simulink model "MATE_SwitchedReluctanceMotor64Drive"  (R2024b)
settings: Solver=FixedStepDiscrete  StartTime=0.0  StopTime=5  FixedStep=Ts  RelTol=1e-3  AbsTol=1e-5  EnableMultiTasking=on
PreLoadFcn:
  | Ts=1e-6;Rsnu=100; Csnu=1e-6;
  | 
  | % Magnetisation characteristic table of the switched Reluctance Motor:
  | % Table elements =  Flux linkage, in Wb.
  | 
  | FluxTable = [
  |     0             0              0             0             0             0
  |     0.3220    0.3050    0.2280    0.1240    0.0220    0.0170
  |     0.3760    0.3570    0.2770    0.1600    0.0420    0.0340
  |     0.3990    0.3850    0.3000    0.1830    0.0640    0.0500
  |     0.4160    0.4020    0.3200    0.2010    0.0840    0.0670
  |     0.4280    0.4150    0.3340    0.2190    0.1030    0.0840
  |     0.4370    0.4260    0.3480    0.2370    0.1230    0.1010
  |     0.4430    0.4330    0.3590    0.2530    0.1420    0.1170
  |     0.4490    0.4390    0.3710    0.2680    0.1610    0.1340
  |     0.4540    0.4440    0.3820    0.2820    0.1790    0.1510
  |     0.4590    0.4490    0.3920    0.2950    0.1970    0.1680
  |     0.4630    0.4530    0.4020    0.3090    0.2140    0.1840
  |     0.4670    0.4570    0.4110    0.3220    0.2310    0.2010
  |     0.4700    0.4620    0.4190    0.3360    0.2460    0.2180
  |     0.4740    0.4650    0.4270    0.3480    0.2610    0.2350
  |     0.4780    0.4690    0.4330    0.3590    0.2770    0.2510
  |     0.4810    0.4730    0.4380    0.3690    0.2910    0.2680
  |     0.4840    0.4770    0.4440    0.3800    0.3050    0.2850
  |     0.4870    0.4790    0.4480    0.3890    0.3200    0.3020];
  | 
  | % Table columns :  Rotor angles, in degrees.
  | 
  | RotorAngles = [
  |     0             10            20            30            40            45];
  | 
  | % Table rows : Stator current, in A.
  | 
  | StatorCurrents = [ 0:size(FluxTable,1)-1] * 25;
PostLoadFcn:
  | Ts=1e-6;Rsnu=100; Csnu=1e-6;
  | 
  | % Magnetisation characteristic table of the switched Reluctance Motor:
  | % Table elements =  Flux linkage, in Wb.
  | 
  | FluxTable = [
  |     0             0              0             0             0             0
  |     0.3220    0.3050    0.2280    0.1240    0.0220    0.0170
  |     0.3760    0.3570    0.2770    0.1600    0.0420    0.0340
  |     0.3990    0.3850    0.3000    0.1830    0.0640    0.0500
  |     0.4160    0.4020    0.3200    0.2010    0.0840    0.0670
  |     0.4280    0.4150    0.3340    0.2190    0.1030    0.0840
  |     0.4370    0.4260    0.3480    0.2370    0.1230    0.1010
  |     0.4430    0.4330    0.3590    0.2530    0.1420    0.1170
  |     0.4490    0.4390    0.3710    0.2680    0.1610    0.1340
  |     0.4540    0.4440    0.3820    0.2820    0.1790    0.1510
  |     0.4590    0.4490    0.3920    0.2950    0.1970    0.1680
  |     0.4630    0.4530    0.4020    0.3090    0.2140    0.1840
  |     0.4670    0.4570    0.4110    0.3220    0.2310    0.2010
  |     0.4700    0.4620    0.4190    0.3360    0.2460    0.2180
  |     0.4740    0.4650    0.4270    0.3480    0.2610    0.2350
  |     0.4780    0.4690    0.4330    0.3590    0.2770    0.2510
  |     0.4810    0.4730    0.4380    0.3690    0.2910    0.2680
  |     0.4840    0.4770    0.4440    0.3800    0.3050    0.2850
  |     0.4870    0.4790    0.4480    0.3890    0.3200    0.3020];
  | 
  | % Table columns :  Rotor angles, in degrees.
  | 
  | RotorAngles = [
  |     0             10            20            30            40            45];
  | 
  | % Table rows : Stator current, in A.
  | 
  | StatorCurrents = [ 0:size(FluxTable,1)-1] * 25;
InitFcn:
  | Ts=1e-6;Rsnu=100; Csnu=1e-6;
  | 
  | % Magnetisation characteristic table of the switched Reluctance Motor:
  | % Table elements =  Flux linkage, in Wb.
  | 
  | FluxTable = [
  |     0             0              0             0             0             0
  |     0.3220    0.3050    0.2280    0.1240    0.0220    0.0170
  |     0.3760    0.3570    0.2770    0.1600    0.0420    0.0340
  |     0.3990    0.3850    0.3000    0.1830    0.0640    0.0500
  |     0.4160    0.4020    0.3200    0.2010    0.0840    0.0670
  |     0.4280    0.4150    0.3340    0.2190    0.1030    0.0840
  |     0.4370    0.4260    0.3480    0.2370    0.1230    0.1010
  |     0.4430    0.4330    0.3590    0.2530    0.1420    0.1170
  |     0.4490    0.4390    0.3710    0.2680    0.1610    0.1340
  |     0.4540    0.4440    0.3820    0.2820    0.1790    0.1510
  |     0.4590    0.4490    0.3920    0.2950    0.1970    0.1680
  |     0.4630    0.4530    0.4020    0.3090    0.2140    0.1840
  |     0.4670    0.4570    0.4110    0.3220    0.2310    0.2010
  |     0.4700    0.4620    0.4190    0.3360    0.2460    0.2180
  |     0.4740    0.4650    0.4270    0.3480    0.2610    0.2350
  |     0.4780    0.4690    0.4330    0.3590    0.2770    0.2510
  |     0.4810    0.4730    0.4380    0.3690    0.2910    0.2680
  |     0.4840    0.4770    0.4440    0.3800    0.3050    0.2850
  |     0.4870    0.4790    0.4480    0.3890    0.3200    0.3020];
  | 
  | % Table columns :  Rotor angles, in degrees.
  | 
  | RotorAngles = [
  |     0             10            20            30            40            45];
  | 
  | % Table rows : Stator current, in A.
  | 
  | StatorCurrents = [ 0:size(FluxTable,1)-1] * 25;
undefined symbols (not defined in the file or in its folder): DiscIntNeverNeededParam
libraries: simetranss x5, fl_lib x3, nesl_utility x2
Description:
  | Copyright 2008-2017 The MathWorks, Inc.
settings Model: ARTEMISmethode_block_infos=$$__separator__$$  Creator=Kyle Diller  LastModifiedBy=CD8435
settings SolverCC: AutoScaleAbsTol=off  AlgebraicLoopSolver=TrustRegion  InsertRTBMode=Auto
settings DataIOCC: LimitDataPoints=on  SaveFormat=Array  SignalLoggingSaveFormat=ModelDataLogs  ReturnWorkspaceOutputs=off  SignalLoggingName=sigsOut
settings OptimizationCC: ExpressionDepthLimit=2147483647  InitFltsAndDblsToZero=on  LifeSpan=inf
settings DebuggingCC: UnderspecifiedInitializationDetection=Classic  MergeDetectMultiDrivingBlocksExec=none  CheckExecutionContextPreStartOutputMsg=on  SignalResolutionControl=TryResolveAllWithWarning  MultiTaskDSMMsg=warning  MultiTaskCondExecSysMsg=none  FcnCallInpInsideContextMsg=warning  UnconnectedInputMsg=warning  UnconnectedOutputMsg=warning  UnconnectedLineMsg=warning  StateNameClashWarn=warning  SFUnexpectedBacktrackingDiag=warning  SFNoUnconditionalDefaultTransitionDiag=warning  SFExecutionAtInitializationDiag=none  ArithmeticOperatorsInVariantConditions=warning
settings HardwareCC: ProdBitPerPointer=32  ProdBitPerSizeT=32  ProdBitPerPtrDiffT=32  ProdLargestAtomicFloat=None  ProdIntDivRoundTo=Undefined  ProdEndianess=Unspecified  ProdWordSize=32  ProdHWDeviceType=32-bit Generic  TargetUnknown=on
settings ModelReferenceCC: EnableRefExpFcnMdlSchedulingChecks=on  PropagateSignalLabelsOutOfModel=off
settings SFSimCC: SimUseLocalCustomCode=off  CustomCodeUndefinedFunction=UseInterfaceOnly
settings RTWCC: RTWUseLocalCustomCode=off  GPUComputeCapability=3.5
settings CodeAppCC: StateflowObjectComments=on
settings GRTTargetCC: TargetLangStandard=C89/C90 (ANSI)  CombineOutputUpdateFcns=off  GRTInterface=on
settings ConfigComp: CovMetricSettings=dw  CovSaveCumulativeToWorkspaceVar=on  CovSaveSingleToWorkspaceVar=on  CovExternalEMLEnable=off  CovSFcnEnable=off
settings SimscapeCC: SimscapeNormalizeSystem=off

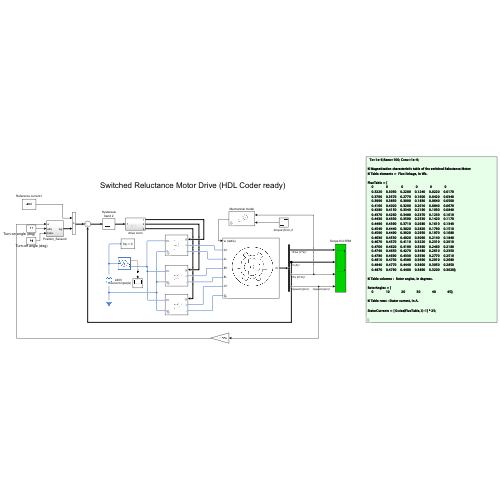
[thumbnail: Simulink's stored preview of the top-level diagram]
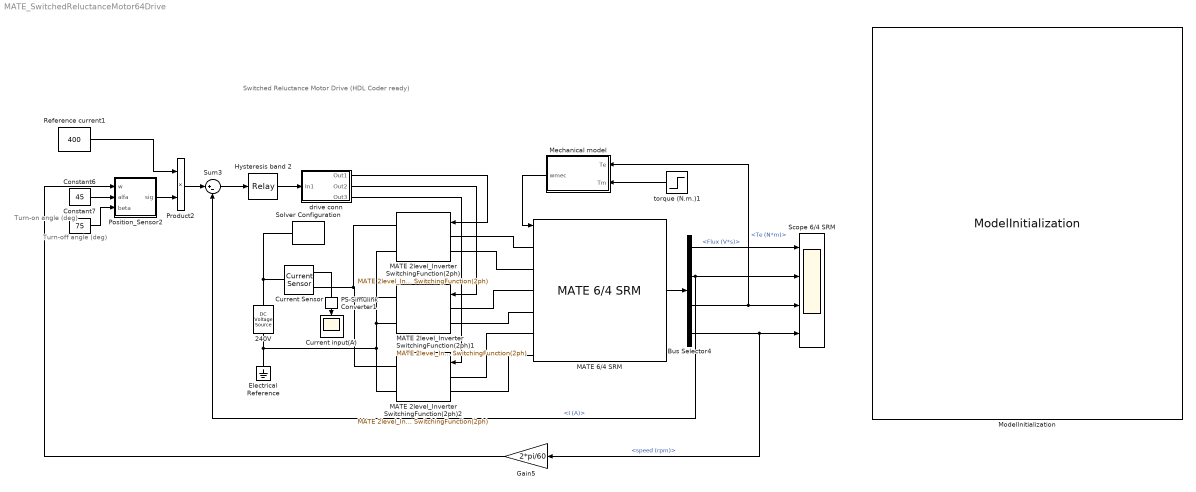
== system MATE_SwitchedReluctanceMotor64Drive ==
  note: Switched Reluctance Motor Drive (HDL Coder ready)
  note: Turn-off angle (deg)
  note: Turn-on angle (deg)
  240V : fl_lib/Electrical/Electrical Sources/DC Voltage Source  v0=240 V
  Bus Selector4 : BusSelector  OutputSignals=Flux (V*s),I (A),Te (N*m),speed (rpm)
  Constant6 : Constant  Value=45
  Constant7 : Constant  Value=75
  Current Sensor : fl_lib/Electrical/Electrical Sensors/Current Sensor
  Current input(A) : Scope
  Electrical Reference : fl_lib/Electrical/Electrical Elements/Electrical Reference
  Gain5 : Gain  Gain=2*pi/60  SaturateOnIntegerOverflow=on  OutDataTypeStr=Inherit: Same as input  ParamDataTypeStr=Inherit: Same as input
  Hysteresis band 2 : Relay  OnSwitchValue=10  OffSwitchValue=-10  SampleTime=Ts
  MATE 2level_Inverter SwitchingFunction(2ph) : simetranss/FPGA/MATE 2level_Inverter  SwitchingFunction(2ph)  Ron=1e-3  Gp=250  Gi=0.1e-6  Ts=Ts  min_charge=0
  MATE 2level_Inverter SwitchingFunction(2ph)1 : simetranss/FPGA/MATE 2level_Inverter  SwitchingFunction(2ph)  Ron=1e-3  Gp=250  Gi=0.1e-6  Ts=Ts  min_charge=0
  MATE 2level_Inverter SwitchingFunction(2ph)2 : simetranss/FPGA/MATE 2level_Inverter  SwitchingFunction(2ph)  Ron=1e-3  Gp=250  Gi=0.1e-6  Ts=Ts  min_charge=0
  MATE 6/4 SRM : simetranss/Machines/MATE 6//4 SRM  MachineType=6/4  Rs=0.05  Inertia=0.05  FluxTable=FluxTable  RotorAngles=RotorAngles  StatorCurrents=StatorCurrents  Friction=0.02  Initialangle=0  TsBlock=-1  nb_points=[100,20,20]  PlotCurves=on
  Mechanical model : Subsystem  mask(Machine rotational mechanical model){J=0.5, F=0.02, fo=0, Ts=Ts}
      mask prompts: J "Inertia (kg.m^2)"; F "Friction (N.m.s)"; fo "Initial mechanical frequency (Hz)"; Ts "Sample Time (s)"
      mask help:
      | This block can implement a simple rotating mechanical equation for machines
      |
      | The block working equation is:
      | wmec=1/J*INT{( Te - Tm -F*wmec )*dt}
      |
      | All values in SI.
      |
      | Parameters:
      | Inertia J (kg.m^2)
      | Friction F (N.m.s)
      | Initial mechanical frequency (Hz)
      | Sample Time (s).
      |
      | Signals:
      | Te: electric torque input from the machine (N.m.)
      | Tm : mechanical torque applied to the shaft (N.m.)
      | wmec: mechanical speed of machine (rad/s)
      |
      | Conversion from Per-Unit values
      |
      | J=2*H*Pn/w_mec^2
      | F=D*Pn/w_mec^2
      | where:
      | J is the inertia in km.m^2
      | H is the inertia constant in seconds.
      | F is the friction factor in N.m.s
      | D in the friction factor or damping factor in pu.
      | Pn is the nominal power of the machine
      | w_mec is the nominal mechanical rotational frequency of the machine in rad/s
  ModelInitialization : simetranss/Usefulls/ModelInitialization  InitFcnX=|  prel=on  posl=on  inif=on  strf=off
      | Ts=1e-6;Rsnu=100; Csnu=1e-6; 
      | 
      | % Magnetisation characteristic table of the switched Reluctance Motor:
      | % Table elements =  Flux linkage, in Wb.
      | 
      | FluxTable = [
      |     0             0              0             0             0             0
      |     0.3220    0.3050    0.2280    0.1240    0.0220    0.0170
      |     0.3760    0.3570    0.2770    0.1600    0.0420    0.0340
      |     0.3990    0.3850    0.3000    0.1830    0.0640    0.0500
      |     0.4160    0.4020    0.3200    0.2010    0.0840    0.0670
      |     0.4280    0.4150    0.3340    0.2190    0.1030    0.0840
      |     0.4370    0.4260    0.3480    0.2370    0.1230    0.1010
      |     0.4430    0.4330    0.3590    0.2530    0.1420    0.1170
      |     0.4490    0.4390    0.3710    0.2680    0.1610    0.1340
      |     0.4540    0.4440    0.3820    0.2820    0.1790    0.1510
      |     0.4590    0.4490    0.3920    0.2950    0.1970    0.1680
      |     0.4630    0.4530    0.4020    0.3090    0.2140    0.1840
      |     0.4670    0.4570    0.4110    0.3220    0.2310    0.2010
      |     0.4700    0.4620    0.4190    0.3360    0.2460    0.2180
      |     0.4740    0.4650    0.4270    0.3480    0.2610    0.2350
      |     0.4780    0.4690    0.4330    0.3590    0.2770    0.2510
      |     0.4810    0.4730    0.4380    0.3690    0.2910    0.2680
      |     0.4840    0.4770    0.4440    0.3800    0.3050    0.2850
      |     0.4870    0.4790    0.4480    0.3890    0.3200    0.3020]; 
      | 
      | % Table columns :  Rotor angles, in degrees.
      | 
      | RotorAngles = [
      |     0             10            20            30            40            45];
      | 
      | % Table rows : Stator current, in A.
      | 
      | StatorCurrents = [ 0:size(FluxTable,1)-1] * 25;
  PS-Simulink Converter1 : nesl_utility/PS-Simulink Converter  PhysicalDomain=network_engine_domain  SubClassName=ps_output  LeftPortType=input  RightPortType=output  PseudoPeriodic=off  Frequencies=[]  VectorFormat=inherit  Unit=inherit  AffineConversion=off
  Position_Sensor2 : Subsystem
  Product2 : Product  SaturateOnIntegerOverflow=on  OutDataTypeStr=Inherit: Same as first input
  Reference current1 : Constant  Value=400
  Scope 6/4 SRM : Scope  NumInputPorts=4
  Solver Configuration : nesl_utility/Solver Configuration  PhysicalDomain=network_engine_domain  SubClassName=solver  LeftPortType=input  RightPortType=generic  Tones=[]  Harmonics=[]  SimulateNoise=off  Profile=off  UseLocalSampling=off  EnableSwitchedLinearOptims=on  FrequencyDomain=off  UseCCode=off  RelTol=0.001  AbsTol=0.001  MinStep=1e-09  ToWorkspace=off  RevertToSquareIcSolve=off  NumHomotopyIterations=100  PhasorMode=off  PhasorModeNumHarmonics=1  ConsistencySolver=NEWTON_XTOL_AFTER_FTOL  IndexReductionMethod=DerivativeReplacement  DoDC=off  ResidualTolerance=1e-09  ConsistencyTolSource=GLOBAL  ConsistencyAbsTol=0.001  ConsistencyRelTol=0.001  ConsistencyTolFactor=0.001  UseLocalSolver=on  LocalSolverChoice=NE_BACKWARD_EULER_ADVANCER  ResolveIndetEquations=on  FunctionEvalNumThread=1  LocalSolverSampleTime=Ts  DoFixedCost=on  MaxNonlinIter=1  MaxModeIter=2  ComputeImpulses=off  ImpulseIterations=2  LinearAlgebra=auto  LinearAlgebraNumThread=0  EquationFormulation=NE_TIME_EF  DelaysMemoryBudget=1024  AutomaticFiltering=on  FilteringTimeConstant=0.001  PartitionStorageMethod=AS_NEEDED  PartitionMemoryBudget=1024  PartitionMethod=ROBUST  MultibodyUseLocalSolver=off  MultibodyLocalSolverChoice=ODE1  MultibodyLocalSolverSampleTime=0.001
  Sum3 : Sum  Inputs=|+-  SaturateOnIntegerOverflow=on
  drive conn : Subsystem
  torque (N.m.)1 : Step  After=100  SampleTime=0
  wires:
  Bus Selector4/3 -> Mechanical model/1(Te), Scope 6/4 SRM/3  "<Te (N*m)>"
  Constant6/1 -> Position_Sensor2/2(alfa)
  Constant7/1 -> Position_Sensor2/3(beta)
  Sum3/1 -> Hysteresis band 2/1
  Product2/1 -> Sum3/1
  Position_Sensor2/1(sig) -> Product2/2
  MATE 6/4 SRM/1 -> Bus Selector4/1
  Bus Selector4/1 -> Scope 6/4 SRM/1  "<Flux (V*s)>"
  Bus Selector4/2 -> Scope 6/4 SRM/2, Sum3/2  "<I (A)>"
  Bus Selector4/4 -> Scope 6/4 SRM/4, Gain5/1  "<speed (rpm)>"
  torque (N.m.)1/1 -> Mechanical model/2(Tm)
  Gain5/1 -> Position_Sensor2/1(w)
  Mechanical model/1(wmec) -> MATE 6/4 SRM/1
  Reference current1/1 -> Product2/1
  drive conn/1(Out1) -> MATE 2level_Inverter SwitchingFunction(2ph)/1
  drive conn/2(Out2) -> MATE 2level_Inverter SwitchingFunction(2ph)1/1
  drive conn/3(Out3) -> MATE 2level_Inverter SwitchingFunction(2ph)2/1
  PS-Simulink Converter1/1 -> Current input(A)/1
  Hysteresis band 2/1 -> drive conn/1(In1)
  connections:
  Solver Configuration/RConn1 -- 240V/LConn1 -- Current Sensor/LConn1
  240V/RConn1 -- MATE 2level_Inverter SwitchingFunction(2ph)2/RConn2 -- MATE 2level_Inverter SwitchingFunction(2ph)1/RConn2 -- MATE 2level_Inverter SwitchingFunction(2ph)/RConn2 -- Electrical Reference/LConn1
  Current Sensor/RConn1 -- PS-Simulink Converter1/LConn1
  MATE 2level_Inverter SwitchingFunction(2ph)2/RConn1 -- MATE 2level_Inverter SwitchingFunction(2ph)1/RConn1 -- MATE 2level_Inverter SwitchingFunction(2ph)/RConn1 -- Current Sensor/RConn2
  MATE 2level_Inverter SwitchingFunction(2ph)/LConn1 -- MATE 6/4 SRM/LConn1
  MATE 2level_Inverter SwitchingFunction(2ph)1/LConn2 -- MATE 6/4 SRM/LConn4
  MATE 2level_Inverter SwitchingFunction(2ph)/LConn2 -- MATE 6/4 SRM/LConn2
  MATE 2level_Inverter SwitchingFunction(2ph)1/LConn1 -- MATE 6/4 SRM/LConn3
  MATE 2level_Inverter SwitchingFunction(2ph)2/LConn2 -- MATE 6/4 SRM/LConn6
  MATE 2level_Inverter SwitchingFunction(2ph)2/LConn1 -- MATE 6/4 SRM/LConn5

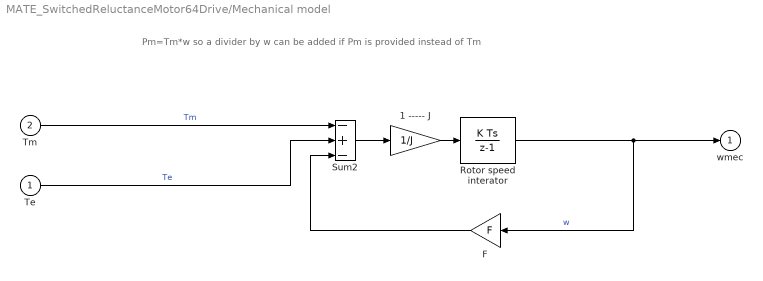
== system MATE_SwitchedReluctanceMotor64Drive/Mechanical model ==
  note: Pm=Tm*w so a divider by w can be added if Pm is provided instead of Tm
  Te : Inport  PortDimensions=1
  Tm : Inport  Port=2
  1 ----- J : Gain  Gain=1/J  SaturateOnIntegerOverflow=on  OutDataTypeStr=Inherit: Same as input  ParamDataTypeStr=Inherit: Same as input
  F : Gain  Gain=F  SaturateOnIntegerOverflow=on  OutDataTypeStr=Inherit: Same as input  ParamDataTypeStr=Inherit: Same as input
  Rotor speed interator : DiscreteIntegrator  InitialCondition=fo*2*pi  SampleTime=Ts  ICPrevOutput=DiscIntNeverNeededParam  ICPrevScaledInput=DiscIntNeverNeededParam
  Sum2 : Sum  Inputs=-+-  InputSameDT=on  SaturateOnIntegerOverflow=on  OutDataTypeStr=Inherit: Same as first input
  wmec : Outport  InitialOutput=0  VectorParamsAs1DForOutWhenUnconnected=off
  wires:
  Tm/1 -> Sum2/1  "Tm"
  Sum2/1 -> 1 ----- J/1
  F/1 -> Sum2/3
  Te/1 -> Sum2/2  "Te"
  1 ----- J/1 -> Rotor speed interator/1
  Rotor speed interator/1 -> wmec/1, F/1  "w"

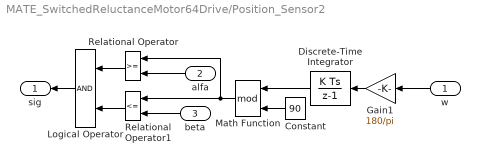
== system MATE_SwitchedReluctanceMotor64Drive/Position_Sensor2 ==
  w : Inport
  alfa : Inport  Port=2
  beta : Inport  Port=3
  Constant : Constant  Value=90
  Discrete-Time Integrator : DiscreteIntegrator  InitialCondition=[0 -30 -60]  SampleTime=Ts  ICPrevOutput=DiscIntNeverNeededParam  ICPrevScaledInput=DiscIntNeverNeededParam
  Gain1 : Gain  Gain=180/pi  SaturateOnIntegerOverflow=on  OutDataTypeStr=Inherit: Same as input  ParamDataTypeStr=Inherit: Same as input
  Logical Operator : Logic  AllPortsSameDT=off
  Math Function : Math  Operator=mod  SignedPower=on
  Relational Operator : RelationalOperator  InputSameDT=off
  Relational Operator1 : RelationalOperator  Operator=<=  InputSameDT=off
  sig : Outport  VectorParamsAs1DForOutWhenUnconnected=off
  wires:
  Logical Operator/1 -> sig/1
  w/1 -> Gain1/1
  Math Function/1 -> Relational Operator/1, Relational Operator1/1
  Relational Operator1/1 -> Logical Operator/2
  Gain1/1 -> Discrete-Time Integrator/1
  beta/1 -> Relational Operator1/2
  alfa/1 -> Relational Operator/2
  Relational Operator/1 -> Logical Operator/1
  Constant/1 -> Math Function/2
  Discrete-Time Integrator/1 -> Math Function/1

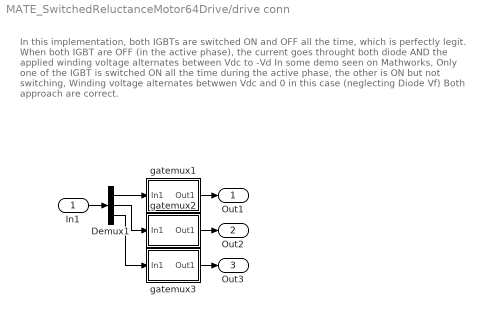
== system MATE_SwitchedReluctanceMotor64Drive/drive conn ==
  note: In this implementation, both IGBTs are switched ON and OFF all the time, which is perfectly legit. When both IGBT are OFF (in the active phase), the current goes throught both diode AND the applied winding voltage alternates between Vdc to -Vd
      |
      | In some demo seen on Mathworks, Only one of the IGBT is switched ON all the time during the active phase, the other is ON but not switching, Winding voltage alternates betwwen Vdc and 0 in this case (neglecting Diode Vf)
      |
      | Both approach are correct.
  In1 : Inport
  Demux1 : Demux  Outputs=3
  gatemux1 : Subsystem
  gatemux2 : Subsystem
  gatemux3 : Subsystem
  Out1 : Outport
  Out2 : Outport  Port=2
  Out3 : Outport  Port=3
  wires:
  Demux1/2 -> gatemux2/1(In1)
  gatemux1/1(Out1) -> Out1/1
  Demux1/1 -> gatemux1/1(In1)
  Demux1/3 -> gatemux3/1(In1)
  gatemux2/1(Out1) -> Out2/1
  gatemux3/1(Out1) -> Out3/1
  In1/1 -> Demux1/1

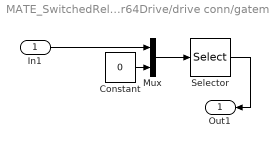
== system MATE_SwitchedReluctanceMotor64Drive/drive conn/gatemux1 ==
  In1 : Inport
  Constant : Constant  Value=0
  Mux : Mux  Inputs=2
  Selector : Selector  InputPortWidth=2  IndexOptions=Index vector (dialog)  Indices=[1 2 2 1]  OutputSizes=1
  Out1 : Outport
  wires:
  Selector/1 -> Out1/1
  In1/1 -> Mux/1
  Mux/1 -> Selector/1
  Constant/1 -> Mux/2

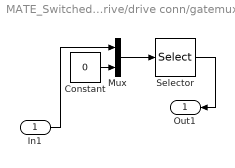
== system MATE_SwitchedReluctanceMotor64Drive/drive conn/gatemux2 ==
  In1 : Inport
  Constant : Constant  Value=0
  Mux : Mux  Inputs=2
  Selector : Selector  InputPortWidth=2  IndexOptions=Index vector (dialog)  Indices=[1 2 2 1]  OutputSizes=1
  Out1 : Outport
  wires:
  Constant/1 -> Mux/2
  Mux/1 -> Selector/1
  In1/1 -> Mux/1
  Selector/1 -> Out1/1

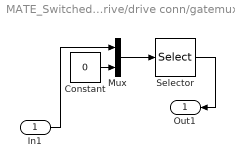
== system MATE_SwitchedReluctanceMotor64Drive/drive conn/gatemux3 ==
  In1 : Inport
  Constant : Constant  Value=0
  Mux : Mux  Inputs=2
  Selector : Selector  InputPortWidth=2  IndexOptions=Index vector (dialog)  Indices=[1 2 2 1]  OutputSizes=1
  Out1 : Outport
  wires:
  Selector/1 -> Out1/1
  In1/1 -> Mux/1
  Mux/1 -> Selector/1
  Constant/1 -> Mux/2
